simulink model "unicycle_cosim"  (R2025b)
settings: Solver=ode1  StartTime=0  StopTime=inf  FixedStep=0.07  RelTol=1e-3
settings Model: Creator=navid  LastModifiedBy=navid
settings DataIOCC: SaveOutput=off  SaveTime=off  ReturnWorkspaceOutputs=off

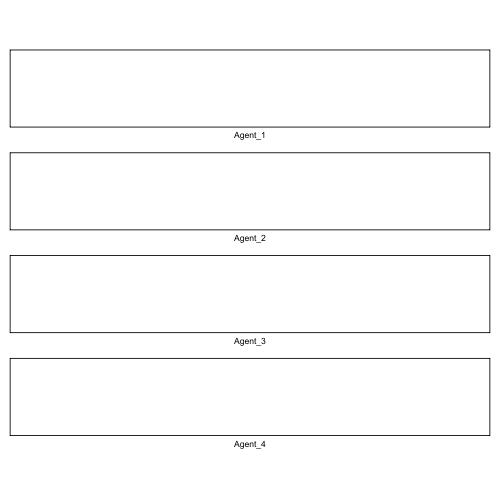
[thumbnail: Simulink's stored preview of the top-level diagram]
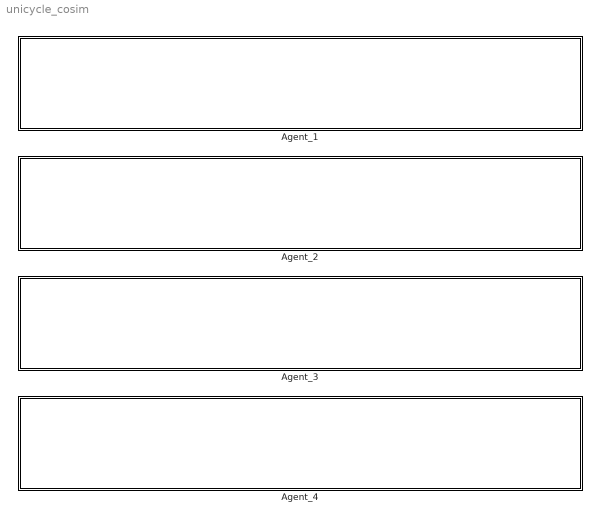
== system unicycle_cosim ==
  Agent_1 : Subsystem
  Agent_2 : Subsystem
  Agent_3 : Subsystem
  Agent_4 : Subsystem

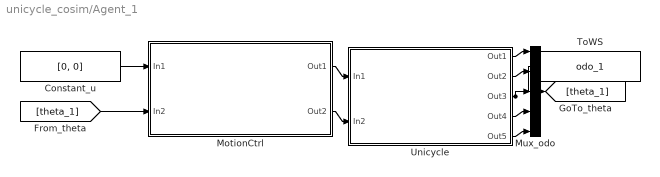
== system unicycle_cosim/Agent_1 ==
  Constant_u : Constant  Value=[0, 0]  SampleTime=0.07
  MotionCtrl : Subsystem
  Mux_odo : Mux  Inputs=5
  ToWS : ToWorkspace  VariableName=odo_1  SampleTime=0.07
  Unicycle : Subsystem
  wires:
  Constant_u/1 -> MotionCtrl/1(In1)
  [theta_1] -> MotionCtrl/2(In2)
  MotionCtrl/1(Out1) -> Unicycle/1(In1)
  MotionCtrl/2(Out2) -> Unicycle/2(In2)
  Unicycle/1(Out1) -> Mux_odo/1
  Unicycle/2(Out2) -> Mux_odo/2
  Unicycle/3(Out3) -> Mux_odo/3, [theta_1]
  Unicycle/4(Out4) -> Mux_odo/4
  Unicycle/5(Out5) -> Mux_odo/5
  Mux_odo/1 -> ToWS/1

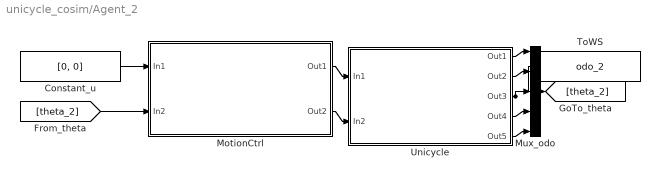
== system unicycle_cosim/Agent_2 ==
  Constant_u : Constant  Value=[0, 0]  SampleTime=0.07
  MotionCtrl : Subsystem
  Mux_odo : Mux  Inputs=5
  ToWS : ToWorkspace  VariableName=odo_2  SampleTime=0.07
  Unicycle : Subsystem
  wires:
  Constant_u/1 -> MotionCtrl/1(In1)
  [theta_2] -> MotionCtrl/2(In2)
  MotionCtrl/1(Out1) -> Unicycle/1(In1)
  MotionCtrl/2(Out2) -> Unicycle/2(In2)
  Unicycle/1(Out1) -> Mux_odo/1
  Unicycle/2(Out2) -> Mux_odo/2
  Unicycle/3(Out3) -> Mux_odo/3, [theta_2]
  Unicycle/4(Out4) -> Mux_odo/4
  Unicycle/5(Out5) -> Mux_odo/5
  Mux_odo/1 -> ToWS/1

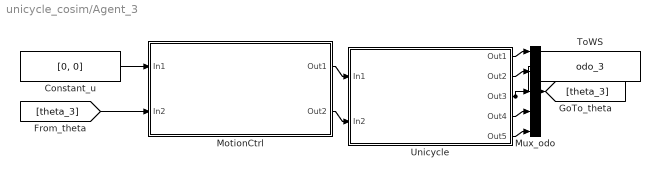
== system unicycle_cosim/Agent_3 ==
  Constant_u : Constant  Value=[0, 0]  SampleTime=0.07
  MotionCtrl : Subsystem
  Mux_odo : Mux  Inputs=5
  ToWS : ToWorkspace  VariableName=odo_3  SampleTime=0.07
  Unicycle : Subsystem
  wires:
  Constant_u/1 -> MotionCtrl/1(In1)
  [theta_3] -> MotionCtrl/2(In2)
  MotionCtrl/1(Out1) -> Unicycle/1(In1)
  MotionCtrl/2(Out2) -> Unicycle/2(In2)
  Unicycle/1(Out1) -> Mux_odo/1
  Unicycle/2(Out2) -> Mux_odo/2
  Unicycle/3(Out3) -> Mux_odo/3, [theta_3]
  Unicycle/4(Out4) -> Mux_odo/4
  Unicycle/5(Out5) -> Mux_odo/5
  Mux_odo/1 -> ToWS/1

== system unicycle_cosim/Agent_4 ==
  Constant_u : Constant  Value=[0, 0]  SampleTime=0.07
  MotionCtrl : Subsystem
  Mux_odo : Mux  Inputs=5
  ToWS : ToWorkspace  VariableName=odo_4  SampleTime=0.07
  Unicycle : Subsystem
  wires:
  Constant_u/1 -> MotionCtrl/1(In1)
  [theta_4] -> MotionCtrl/2(In2)
  MotionCtrl/1(Out1) -> Unicycle/1(In1)
  MotionCtrl/2(Out2) -> Unicycle/2(In2)
  Unicycle/1(Out1) -> Mux_odo/1
  Unicycle/2(Out2) -> Mux_odo/2
  Unicycle/3(Out3) -> Mux_odo/3, [theta_4]
  Unicycle/4(Out4) -> Mux_odo/4
  Unicycle/5(Out5) -> Mux_odo/5
  Mux_odo/1 -> ToWS/1

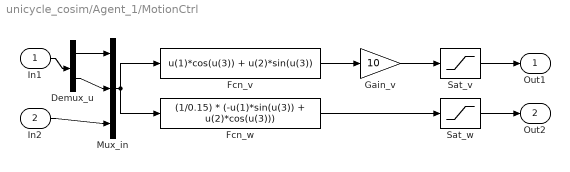
== system unicycle_cosim/Agent_1/MotionCtrl ==
  In1 : Inport
  In2 : Inport  Port=2
  Demux_u : Demux  Outputs=2
  Fcn_v : Fcn  Expr=u(1)*cos(u(3)) + u(2)*sin(u(3))
  Fcn_w : Fcn  Expr=(1/0.15) * (-u(1)*sin(u(3)) + u(2)*cos(u(3)))
  Gain_v : Gain  Gain=10
  Mux_in : Mux  Inputs=3
  Sat_v : Saturate  UpperLimit=2  LowerLimit=-2
  Sat_w : Saturate  UpperLimit=6  LowerLimit=-6
  Out1 : Outport
  Out2 : Outport  Port=2
  wires:
  In1/1 -> Demux_u/1
  Demux_u/1 -> Mux_in/1
  Demux_u/2 -> Mux_in/2
  In2/1 -> Mux_in/3
  Mux_in/1 -> Fcn_v/1, Fcn_w/1
  Fcn_v/1 -> Gain_v/1
  Gain_v/1 -> Sat_v/1
  Fcn_w/1 -> Sat_w/1
  Sat_v/1 -> Out1/1
  Sat_w/1 -> Out2/1

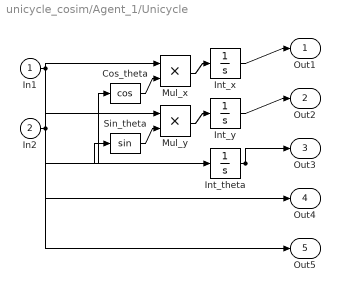
== system unicycle_cosim/Agent_1/Unicycle ==
  In1 : Inport
  In2 : Inport  Port=2
  Cos_theta : Trigonometry  Operator=cos
  Int_theta : Integrator
  Int_x : Integrator
  Int_y : Integrator
  Mul_x : Product  Inputs=**
  Mul_y : Product  Inputs=**
  Sin_theta : Trigonometry
  Out1 : Outport
  Out2 : Outport  Port=2
  Out3 : Outport  Port=3
  Out4 : Outport  Port=4
  Out5 : Outport  Port=5
  wires:
  In2/1 -> Int_theta/1, Out5/1
  Int_theta/1 -> Cos_theta/1, Sin_theta/1, Out3/1
  Cos_theta/1 -> Mul_x/2
  In1/1 -> Mul_x/1, Mul_y/1, Out4/1
  Mul_x/1 -> Int_x/1
  Sin_theta/1 -> Mul_y/2
  Mul_y/1 -> Int_y/1
  Int_x/1 -> Out1/1
  Int_y/1 -> Out2/1

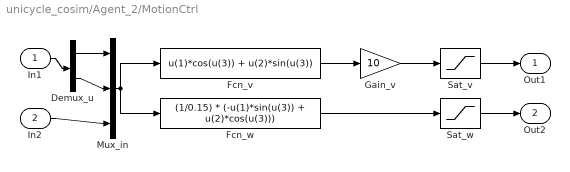
== system unicycle_cosim/Agent_2/MotionCtrl ==
  In1 : Inport
  In2 : Inport  Port=2
  Demux_u : Demux  Outputs=2
  Fcn_v : Fcn  Expr=u(1)*cos(u(3)) + u(2)*sin(u(3))
  Fcn_w : Fcn  Expr=(1/0.15) * (-u(1)*sin(u(3)) + u(2)*cos(u(3)))
  Gain_v : Gain  Gain=10
  Mux_in : Mux  Inputs=3
  Sat_v : Saturate  UpperLimit=2  LowerLimit=-2
  Sat_w : Saturate  UpperLimit=6  LowerLimit=-6
  Out1 : Outport
  Out2 : Outport  Port=2
  wires:
  In1/1 -> Demux_u/1
  Demux_u/1 -> Mux_in/1
  Demux_u/2 -> Mux_in/2
  In2/1 -> Mux_in/3
  Mux_in/1 -> Fcn_v/1, Fcn_w/1
  Fcn_v/1 -> Gain_v/1
  Gain_v/1 -> Sat_v/1
  Fcn_w/1 -> Sat_w/1
  Sat_v/1 -> Out1/1
  Sat_w/1 -> Out2/1

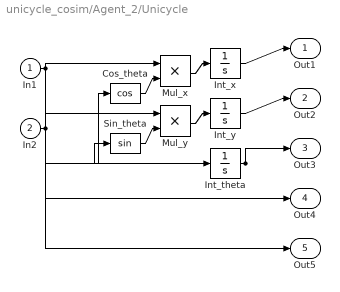
== system unicycle_cosim/Agent_2/Unicycle ==
  In1 : Inport
  In2 : Inport  Port=2
  Cos_theta : Trigonometry  Operator=cos
  Int_theta : Integrator
  Int_x : Integrator
  Int_y : Integrator
  Mul_x : Product  Inputs=**
  Mul_y : Product  Inputs=**
  Sin_theta : Trigonometry
  Out1 : Outport
  Out2 : Outport  Port=2
  Out3 : Outport  Port=3
  Out4 : Outport  Port=4
  Out5 : Outport  Port=5
  wires:
  In2/1 -> Int_theta/1, Out5/1
  Int_theta/1 -> Cos_theta/1, Sin_theta/1, Out3/1
  Cos_theta/1 -> Mul_x/2
  In1/1 -> Mul_x/1, Mul_y/1, Out4/1
  Mul_x/1 -> Int_x/1
  Sin_theta/1 -> Mul_y/2
  Mul_y/1 -> Int_y/1
  Int_x/1 -> Out1/1
  Int_y/1 -> Out2/1

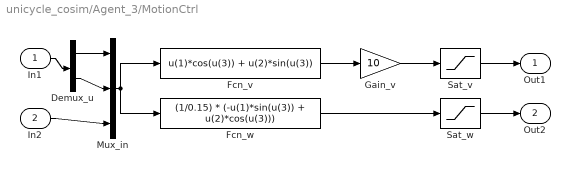
== system unicycle_cosim/Agent_3/MotionCtrl ==
  In1 : Inport
  In2 : Inport  Port=2
  Demux_u : Demux  Outputs=2
  Fcn_v : Fcn  Expr=u(1)*cos(u(3)) + u(2)*sin(u(3))
  Fcn_w : Fcn  Expr=(1/0.15) * (-u(1)*sin(u(3)) + u(2)*cos(u(3)))
  Gain_v : Gain  Gain=10
  Mux_in : Mux  Inputs=3
  Sat_v : Saturate  UpperLimit=2  LowerLimit=-2
  Sat_w : Saturate  UpperLimit=6  LowerLimit=-6
  Out1 : Outport
  Out2 : Outport  Port=2
  wires:
  In1/1 -> Demux_u/1
  Demux_u/1 -> Mux_in/1
  Demux_u/2 -> Mux_in/2
  In2/1 -> Mux_in/3
  Mux_in/1 -> Fcn_v/1, Fcn_w/1
  Fcn_v/1 -> Gain_v/1
  Gain_v/1 -> Sat_v/1
  Fcn_w/1 -> Sat_w/1
  Sat_v/1 -> Out1/1
  Sat_w/1 -> Out2/1

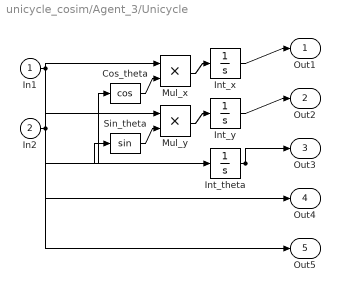
== system unicycle_cosim/Agent_3/Unicycle ==
  In1 : Inport
  In2 : Inport  Port=2
  Cos_theta : Trigonometry  Operator=cos
  Int_theta : Integrator
  Int_x : Integrator
  Int_y : Integrator
  Mul_x : Product  Inputs=**
  Mul_y : Product  Inputs=**
  Sin_theta : Trigonometry
  Out1 : Outport
  Out2 : Outport  Port=2
  Out3 : Outport  Port=3
  Out4 : Outport  Port=4
  Out5 : Outport  Port=5
  wires:
  In2/1 -> Int_theta/1, Out5/1
  Int_theta/1 -> Cos_theta/1, Sin_theta/1, Out3/1
  Cos_theta/1 -> Mul_x/2
  In1/1 -> Mul_x/1, Mul_y/1, Out4/1
  Mul_x/1 -> Int_x/1
  Sin_theta/1 -> Mul_y/2
  Mul_y/1 -> Int_y/1
  Int_x/1 -> Out1/1
  Int_y/1 -> Out2/1

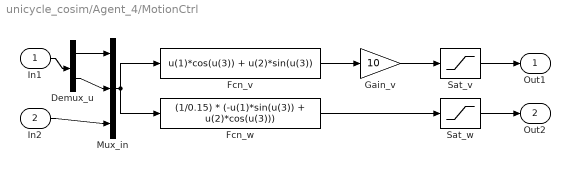
== system unicycle_cosim/Agent_4/MotionCtrl ==
  In1 : Inport
  In2 : Inport  Port=2
  Demux_u : Demux  Outputs=2
  Fcn_v : Fcn  Expr=u(1)*cos(u(3)) + u(2)*sin(u(3))
  Fcn_w : Fcn  Expr=(1/0.15) * (-u(1)*sin(u(3)) + u(2)*cos(u(3)))
  Gain_v : Gain  Gain=10
  Mux_in : Mux  Inputs=3
  Sat_v : Saturate  UpperLimit=2  LowerLimit=-2
  Sat_w : Saturate  UpperLimit=6  LowerLimit=-6
  Out1 : Outport
  Out2 : Outport  Port=2
  wires:
  In1/1 -> Demux_u/1
  Demux_u/1 -> Mux_in/1
  Demux_u/2 -> Mux_in/2
  In2/1 -> Mux_in/3
  Mux_in/1 -> Fcn_v/1, Fcn_w/1
  Fcn_v/1 -> Gain_v/1
  Gain_v/1 -> Sat_v/1
  Fcn_w/1 -> Sat_w/1
  Sat_v/1 -> Out1/1
  Sat_w/1 -> Out2/1

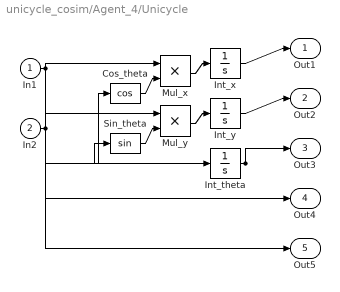
== system unicycle_cosim/Agent_4/Unicycle ==
  In1 : Inport
  In2 : Inport  Port=2
  Cos_theta : Trigonometry  Operator=cos
  Int_theta : Integrator
  Int_x : Integrator
  Int_y : Integrator
  Mul_x : Product  Inputs=**
  Mul_y : Product  Inputs=**
  Sin_theta : Trigonometry
  Out1 : Outport
  Out2 : Outport  Port=2
  Out3 : Outport  Port=3
  Out4 : Outport  Port=4
  Out5 : Outport  Port=5
  wires:
  In2/1 -> Int_theta/1, Out5/1
  Int_theta/1 -> Cos_theta/1, Sin_theta/1, Out3/1
  Cos_theta/1 -> Mul_x/2
  In1/1 -> Mul_x/1, Mul_y/1, Out4/1
  Mul_x/1 -> Int_x/1
  Sin_theta/1 -> Mul_y/2
  Mul_y/1 -> Int_y/1
  Int_x/1 -> Out1/1
  Int_y/1 -> Out2/1
